simulink model "assignment1"  (R2018a)
settings: Solver=VariableStepAuto  StartTime=0.0  StopTime=500  RelTol=1e-3
libraries: simulink x1
settings Model: Creator=krman  LastModifiedBy=Aniket Raj

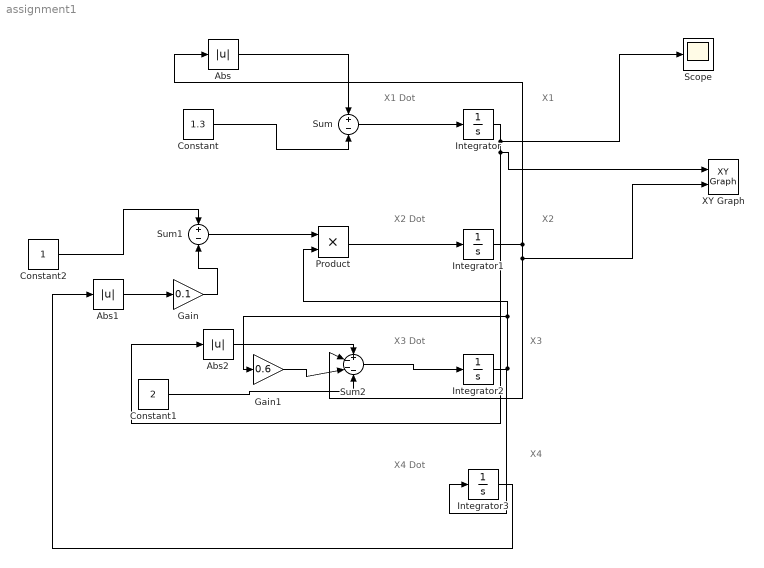
== system assignment1 ==
  note: X1 Dot
  note: X2 Dot
  note: X3 Dot
  note: X4 Dot
  note: X1
  note: X2
  note: X3
  note: X4
  Abs : Abs
  Abs1 : Abs
  Abs2 : Abs
  Constant : Constant  Value=1.3
  Constant1 : Constant  Value=2
  Constant2 : Constant
  Gain : Gain  Gain=0.1
  Gain1 : Gain  Gain=0.6
  Integrator{,1..3} (4 alike) : Integrator  InitialCondition=1
  Product : Product
  Scope : Scope
  Sum : Sum  Inputs=+-
  Sum1 : Sum  Inputs=+-
  Sum2 : Sum  Inputs=+---
  XY Graph : simulink/Sinks/XY Graph  xmin=-50  xmax=50  ymin=-50  ymax=50  st=0.01
  wires:
  Sum/1 -> Integrator/1
  Constant/1 -> Sum/2
  Abs/1 -> Sum/1
  Integrator1/1 -> XY Graph/2, Sum2/2, Abs/1
  Product/1 -> Integrator1/1
  Integrator2/1 -> Integrator3/1, Gain1/1, Product/2
  Sum1/1 -> Product/1
  Constant2/1 -> Sum1/1
  Abs1/1 -> Gain/1
  Gain/1 -> Sum1/2
  Integrator3/1 -> Abs1/1
  Abs2/1 -> Sum2/1
  Integrator/1 -> Scope/1, XY Graph/1, Abs2/1
  Gain1/1 -> Sum2/3
  Constant1/1 -> Sum2/4
  Sum2/1 -> Integrator2/1
